simulink model "Model12016a"  (Simulink 8.8)
settings: Solver=VariableStepAuto  StartTime=0.0  StopTime=100  RelTol=1e-3
values from neighbouring files (symbols this model uses):
  A = M3*(-M1'*M1+(M2-M2'))/M3    [sysgen.m]
  B = randn(n,nu)    [sysgen.m]
  Bd = rand(n,nd)    [sysgen.m]
  C = randn(ny,n)    [sysgen.m]
  Cz = randn(nz,n)    [sysgen.m]
  D = zeros(m,m,2^m)    [faultsgen.m]    (also in sysgen.m = zeros(nz,nd); testScript.m = Delta(:,:,iFFTC))
  Dd = rand(ny,nd)    [sysgen.m]
  K = K_FFTC    [testScript.m]
  L = L_FFTC    [testScript.m]
undefined symbols (not defined in the file or in its folder): DH
settings Model: Creator=vk1014  LastModifiedBy=kc
settings DataIOCC: LimitDataPoints=off  SaveFormat=Dataset  SignalLoggingSaveFormat=Dataset
settings DebuggingCC: UnderspecifiedInitializationDetection=Simplified  MergeDetectMultiDrivingBlocksExec=error  FcnCallInpInsideContextMsg=error  StateNameClashWarn=none  SFUnexpectedBacktrackingDiag=error  SFNoUnconditionalDefaultTransitionDiag=error
settings HardwareCC: ProdBitPerPointer=64  ProdBitPerSizeT=64  ProdBitPerPtrDiffT=64  ProdLargestAtomicFloat=Float  ProdIntDivRoundTo=Zero  ProdEndianess=LittleEndian  ProdWordSize=64  ProdHWDeviceType=Intel->x86-64 (Windows64)
settings ModelReferenceCC: PropagateSignalLabelsOutOfModel=on
settings GRTTargetCC: TargetLangStandard=C99 (ISO)  GeneratePreprocessorConditionals=Use local settings  CombineOutputUpdateFcns=on  GRTInterface=off
settings ConfigComp: CovMetricSettings=dwe  CovHtmlReporting=off  CovSaveCumulativeToWorkspaceVar=off  CovSaveSingleToWorkspaceVar=off  CovExternalEMLEnable=on

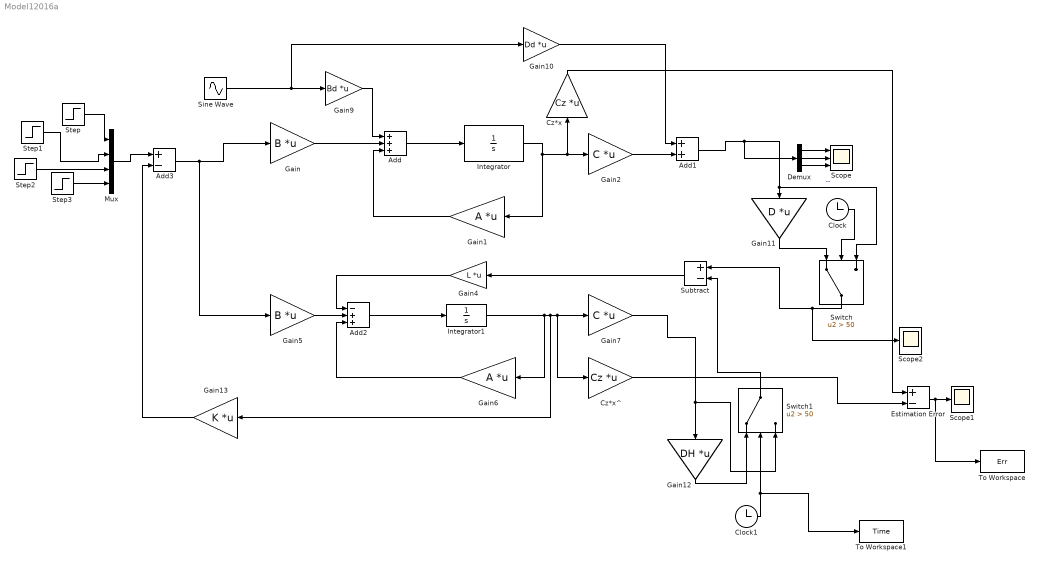
== system Model12016a ==
  Add : Sum  Inputs=+++
  Add1 : Sum
  Add2 : Sum  Inputs=-++
  Add3 : Sum  Inputs=+-
  Clock : Clock
  Clock1 : Clock
  Cz*x : Gain  Gain=Cz  Multiplication=Matrix(K*u)
  Cz*x^ : Gain  Gain=Cz  Multiplication=Matrix(K*u)
  Demux : Demux  Outputs=3
  Estimation Error : Sum  Inputs=+-
  Gain : Gain  Gain=B  Multiplication=Matrix(K*u)
  Gain1 : Gain  Gain=A  Multiplication=Matrix(K*u)
  Gain10 : Gain  Gain=Dd  Multiplication=Matrix(K*u)
  Gain11 : Gain  Gain=D  Multiplication=Matrix(K*u)
  Gain12 : Gain  Gain=DH  Multiplication=Matrix(K*u)
  Gain13 : Gain  Gain=K  Multiplication=Matrix(K*u)
  Gain2 : Gain  Gain=C  Multiplication=Matrix(K*u)
  Gain4 : Gain  Gain=L  Multiplication=Matrix(K*u)
  Gain5 : Gain  Gain=B  Multiplication=Matrix(K*u)
  Gain6 : Gain  Gain=A  Multiplication=Matrix(K*u)
  Gain7 : Gain  Gain=C  Multiplication=Matrix(K*u)
  Gain9 : Gain  Gain=Bd  Multiplication=Matrix(K*u)
  Integrator : Integrator  InitialCondition=1
  Integrator1 : Integrator
  Mux : Mux
  Scope : Scope  NumInputPorts=3
  Scope1 : Scope
  Scope2 : Scope
  Sine Wave : Sin  Amplitude=0.1  SampleTime=0
  Step{,1..3} (4 alike) : Step  SampleTime=0
  Subtract : Sum  Inputs=+-
  Switch : Switch  Criteria=u2 > Threshold  Threshold=50
  Switch1 : Switch  Criteria=u2 > Threshold  Threshold=50
  To Workspace : ToWorkspace  VariableName=Err  SampleTime=-1
      settings: Save2DSignal=2-D array (concatenate along first dimension)
  To Workspace1 : ToWorkspace  VariableName=Time  SampleTime=-1
      settings: Save2DSignal=2-D array (concatenate along first dimension)
  wires:
  Add/1 -> Integrator/1
  Gain/1 -> Add/2
  Integrator/1 -> Cz*x/1, Gain2/1, Gain1/1
  Gain1/1 -> Add/3
  Gain2/1 -> Add1/2
  Add1/1 -> Demux/1, Switch/3, Gain11/1  "--"
  Subtract/1 -> Gain4/1
  Add2/1 -> Integrator1/1
  Gain5/1 -> Add2/2
  Gain6/1 -> Add2/3
  Gain4/1 -> Add2/1
  Integrator1/1 -> Gain6/1, Gain13/1, Cz*x^/1, Gain7/1
  Gain7/1 -> Switch1/3, Gain12/1
  Cz*x/1 -> Estimation Error/1
  Gain9/1 -> Add/1
  Sine Wave/1 -> Gain10/1, Gain9/1
  Gain10/1 -> Add1/1
  Step/1 -> Mux/1
  Step1/1 -> Mux/2
  Step2/1 -> Mux/3
  Step3/1 -> Mux/4
  Demux/2 -> Scope/2
  Demux/1 -> Scope/1
  Demux/3 -> Scope/3
  Cz*x^/1 -> Estimation Error/2
  Clock/1 -> Switch/2
  Switch/1 -> Scope2/1, Subtract/1
  Gain11/1 -> Switch/1
  Clock1/1 -> To Workspace1/1, Switch1/2
  Gain12/1 -> Switch1/1
  Switch1/1 -> Subtract/2
  Add3/1 -> Gain5/1, Gain/1
  Mux/1 -> Add3/1
  Gain13/1 -> Add3/2
  Estimation Error/1 -> To Workspace/1, Scope1/1
